simulink model "SMCEqFinalSim"  (R2024a)
settings: Solver=VariableStepAuto  StartTime=0.0  StopTime=10.0  RelTol=1e-3
undefined symbols (not defined in the file): a, betaF, BetaF, g, J, Kf, Km, Lb, Lm, m_b, m_m
settings Model: Creator=Cami  LastModifiedBy=Cami

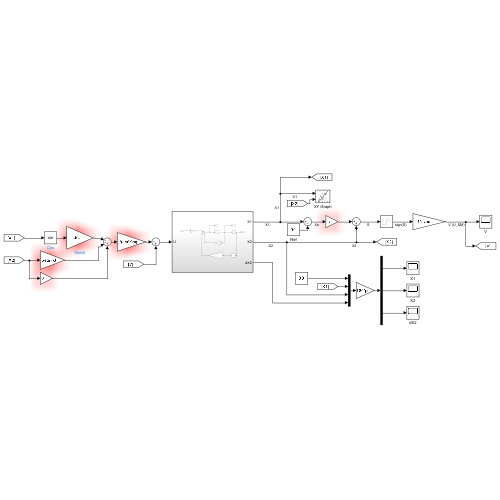
[thumbnail: Simulink's stored preview of the top-level diagram]
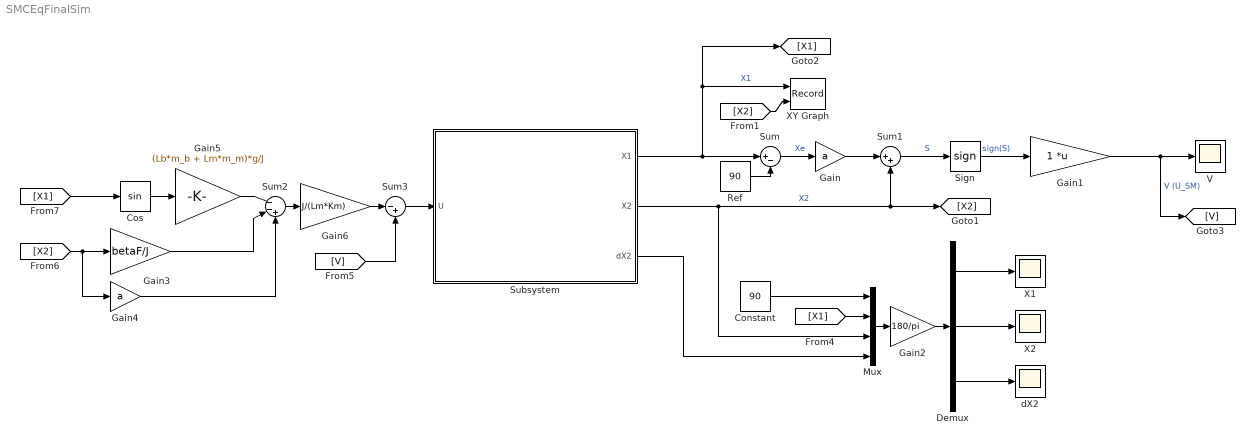
== system SMCEqFinalSim ==
  Constant : Constant  Value=90
  Cos : Trigonometry
  Demux : Demux  Outputs=3
  Gain : Gain  Gain=a
  Gain1 : Gain  Multiplication=Matrix(K*u) (u vector)
  Gain2 : Gain  Gain=180/pi
  Gain3 : Gain  Gain=betaF/J
  Gain4 : Gain  Gain=a
  Gain5 : Gain  Gain=(Lb*m_b + Lm*m_m)*g/J
  Gain6 : Gain  Gain=J/(Lm*Km)
  Mux : Mux
  Ref : Constant  Value=90
  Sign : Signum  ZeroCross=off
  Subsystem : Subsystem
  Sum : Sum  Inputs=|+-
  Sum1 : Sum  Inputs=|++
  Sum2 : Sum  Inputs=|--+
  Sum3 : Sum  Inputs=|-+
  V : Scope
  X1 : Scope
  X2 : Scope
  XY Graph : Record  FileSettingsInternal="{\"entries\":[{\"content\":{\"excelSettings\":{\"content\":{},\"type\":\"Streamout.ExcelSettings\"}},\"type\":\"Streamout.FileSettingStorage\",\"uuid\":\"\"}],\"packageUris\":[\"http:\\/\\/schema.mathworks.com\\/mf0\\/streamout_blocks\\/R2020a\"],\"version\":\"1.0\"}"  Layout=[1 1]  SignalsInternal="{\"entries\":[{\"content\":{\"signals\":[{\"content\":{\"blockPath\":[],\"dimensions\":[1],\"domain\":\"\",\"lineColor\":\"#a2142f\",\"lineWidth\":2,\"plots\":[ 1 ],\"port\":1,\"signalID\":1,\"signalName\":\"X1\"},\"type\":\"RecordBlkView.Signal\",\"uuid\":\"\"},{\"content\":{\"blockPath\":[],\"dimensions\":[1],\"domain\":\"\",\"lineColor\":\"#139fff\",\"lineWidth\":2,\"plots\":[ 1 ],\"port\":2,\"signalID\":2,\"signalName\":\"From1\"},\"type\":\"RecordBlkView.Signal\",\"uuid\":\"\"}]},\"type\":\"RecordBlkView.InputSignals\",\"uuid\":\"\"}],\"packageUris\":[\"http:\\/\\/schema.mathworks.com\\/mf0\\/streamout_blocks\\/R2020a\"],\"version\":\"1.0\"}"  VisualizationBindings="{\"xyplotplugin\":{\"info\":[{\"series\":[{\"bindingParametersList\":[{\"parameter\":\"X-Axis\",\"signalID\":1,\"signalName\":\"X1\"},{\"parameter\":\"Y-Axis\",\"signalID\":2,\"signalName\":\"From1\"}],\"seriesID\":0}],\"subplotID\":1}]}}"  CompatibilityTag=XY
  dX2 : Scope
  wires:
  [X1] -> Cos/1
  Gain3/1 -> Sum2/2
  Constant/1 -> Mux/1
  Ref/1 -> Sum/2
  Demux/2 -> X2/1
  Cos/1 -> Gain5/1
  Gain6/1 -> Sum3/1
  Sum2/1 -> Gain6/1
  [X2] -> Gain4/1, Gain3/1
  Subsystem/3(dX2) -> Mux/4
  Gain5/1 -> Sum2/1
  [V] -> Sum3/2
  Sign/1 -> Gain1/1  "sign(S)"
  Gain2/1 -> Demux/1
  Demux/3 -> dX2/1
  Gain1/1 -> [V], V/1  "V (U_SM)"
  Subsystem/2(X2) -> [X2], Sum1/2, Mux/3  "X2"
  [X1] -> Mux/2
  Subsystem/1(X1) -> Sum/1, [X1], XY Graph/1  "X1"
  [X2] -> XY Graph/2
  Sum3/1 -> Subsystem/1(U)
  Sum/1 -> Gain/1  "Xe"
  Gain/1 -> Sum1/1
  Sum1/1 -> Sign/1  "S"
  Demux/1 -> X1/1
  Gain4/1 -> Sum2/3
  Mux/1 -> Gain2/1

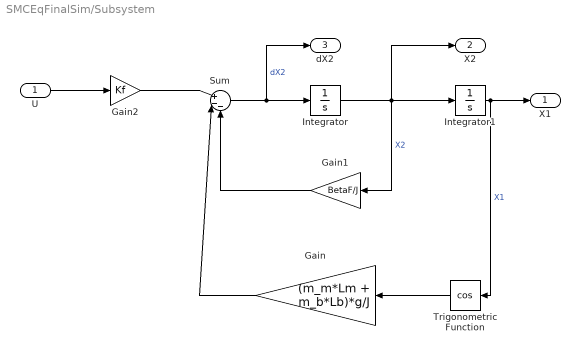
== system SMCEqFinalSim/Subsystem ==
  U : Inport
  Gain : Gain  Gain=(m_m*Lm + m_b*Lb)*g/J
  Gain1 : Gain  Gain=BetaF/J
  Gain2 : Gain  Gain=Kf
  Integrator : Integrator
  Integrator1 : Integrator
  Sum : Sum  Inputs=|+--
  Trigonometric Function : Trigonometry  Operator=cos
  X1 : Outport
  X2 : Outport  Port=2
  dX2 : Outport  Port=3
  wires:
  U/1 -> Gain2/1
  Gain1/1 -> Sum/3
  Gain/1 -> Sum/2
  Gain2/1 -> Sum/1
  Integrator1/1 -> X1/1, Trigonometric Function/1  "X1"
  Trigonometric Function/1 -> Gain/1
  Sum/1 -> dX2/1, Integrator/1  "dX2"
  Integrator/1 -> X2/1, Gain1/1, Integrator1/1  "X2"
